simulink model "Example"  (R2015a)
settings: Solver=ode45  StartTime=0.0  StopTime=inf  RelTol=1e-3
libraries: Joymex2_lib x1
settings Model: Creator=rshu  LastModifiedBy=rshu

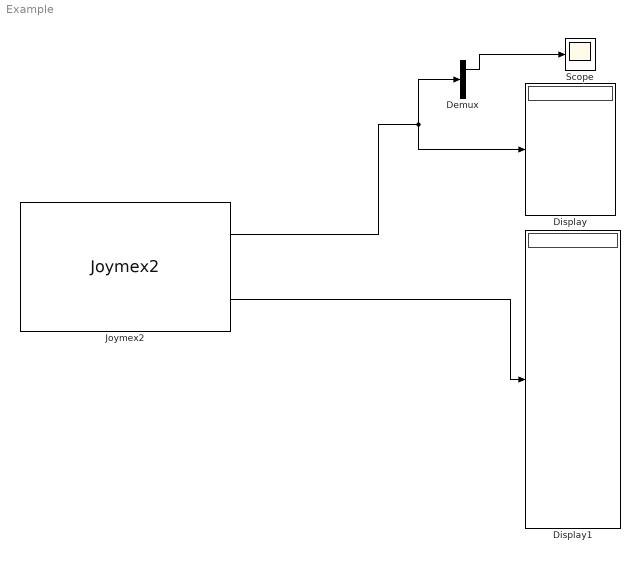
== system Example ==
  Demux : Demux  Outputs=2
  Display : Display
      settings: Decimation=4
  Display1 : Display
  Joymex2 : Joymex2_lib/Joymex2
  Scope : Scope
      settings: YMin=-5000  YMax=35000
  wires:
  Joymex2/2 -> Display1/1
  Joymex2/1 -> Demux/1, Display/1
  Demux/1 -> Scope/1
